simulink model "TDMUX"  (R2021a)
settings: Solver=VariableStepAuto  StartTime=0.0  StopTime=10.0  RelTol=1e-3
values from neighbouring files (symbols this model uses):
  Fs = max(Fs1, Fs2)    [TRY2.m]
libraries: dspsnks4 x1
settings Model: Creator=User  LastModifiedBy=User

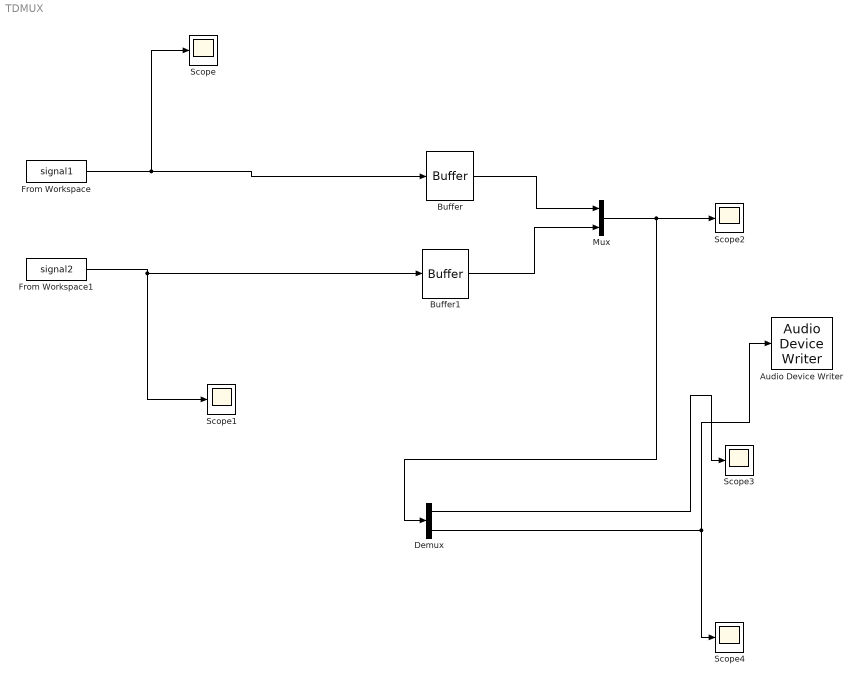
== system TDMUX ==
  Audio Device Writer : dspsnks4/Audio Device Writer  Driver=DirectSound  Device=Default  InheritSampleRate=on  SampleRate=44100  BitDepth=16-bit integer  BufferSize=4096  NumBuffers=10  DefaultOutputChannelMapping=on  OutputChannelMapping=1:2  OutputNumUnderrunSamples=off  DriverIdx=1  DeviceWarnFlag=''
  Buffer : Buffer  N=100  OutputFrames=off
  Buffer1 : Buffer  N=100  OutputFrames=off
  Demux : Demux  Outputs=2
  From Workspace : FromWorkspace  VariableName=signal1  SampleTime=1/Fs
  From Workspace1 : FromWorkspace  VariableName=signal2  SampleTime=1/Fs
  Mux : Mux  Inputs=2
  Scope{,1..4} (5 alike) : Scope
  wires:
  From Workspace/1 -> Buffer/1, Scope/1
  From Workspace1/1 -> Buffer1/1, Scope1/1
  Buffer/1 -> Mux/1
  Buffer1/1 -> Mux/2
  Mux/1 -> Demux/1, Scope2/1
  Demux/1 -> Scope3/1
  Demux/2 -> Scope4/1, Audio Device Writer/1
